simulink model "Motor_Position_Control"  (R2020b)
settings: Solver=VariableStepAuto  StartTime=0.0  StopTime=10.0  RelTol=1e-3
undefined symbols (not defined in the file or in its folder): b, J, Ke, Kt, L, R
settings Model: DataDictionary=values.sldd  Creator=shubham sharma  LastModifiedBy=shubham sharma

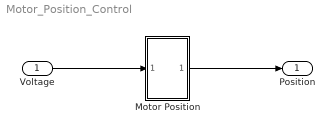
== system Motor_Position_Control ==
  Voltage : Inport
  Motor Position : Subsystem
  Position : Outport
  wires:
  Voltage/1 -> Motor Position/1(In1)
  Motor Position/1(theta) -> Position/1

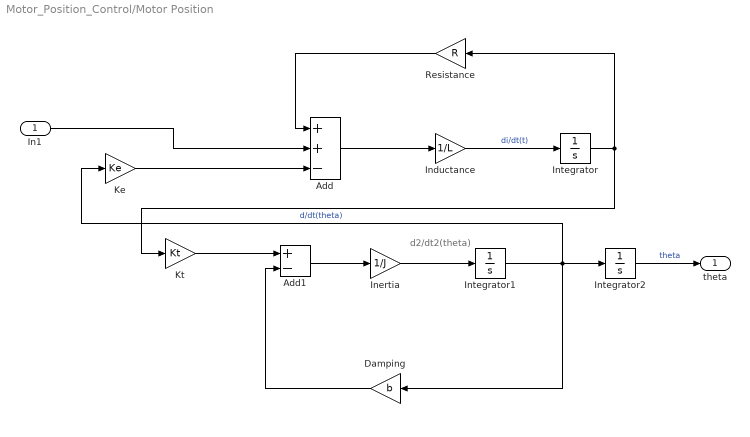
== system Motor_Position_Control/Motor Position ==
  note: d2/dt2(theta)
  In1 : Inport
  Add : Sum  Inputs=++-
  Add1 : Sum  Inputs=+-
  Damping : Gain  Gain=b
  Inductance : Gain  Gain=1/L
  Inertia : Gain  Gain=1/J
  Integrator : Integrator
  Integrator1 : Integrator
  Integrator2 : Integrator
  Ke : Gain  Gain=Ke
  Kt : Gain  Gain=Kt
  Resistance : Gain  Gain=R
  theta : Outport
  wires:
  Integrator/1 -> Kt/1, Resistance/1
  Add1/1 -> Inertia/1
  Inertia/1 -> Integrator1/1
  Kt/1 -> Add1/1
  Damping/1 -> Add1/2
  Inductance/1 -> Integrator/1  "di/dt(t)"
  Integrator2/1 -> theta/1  "theta"
  Resistance/1 -> Add/1
  Add/1 -> Inductance/1
  Integrator1/1 -> Ke/1, Damping/1, Integrator2/1  "d/dt(theta)"
  Ke/1 -> Add/3
  In1/1 -> Add/2
